simulink model "BasicAudio_TranslationEngine64"  (R2022b)
settings: Solver=FixedStepDiscrete  StartTime=0.0  StopTime=5  RelTol=1e-3  EnableMultiTasking=on
InitFcn:
  | % Initialize model
  | run([ ModelRootName() 'Init.m' ]);
  | 
  | % load library data
  | GainLibrary_data;
  | % Load saved values from partition process
  | CapturedConstMask.LoadMapFromFile(bdroot)
model workspace (MAT data in the model file):
  PreampVolumeTable_Idx : Simulink.Signal (value not decoded)
  Range : Simulink.Signal (value not decoded)
  Table_Idx : Simulink.Signal (value not decoded)
undefined symbols (not defined in the file or in its folder): Row
libraries: TuneVar x50, TOP x27, FeaturePath x7, CapturedConstLib x3
(part 2 of 4)

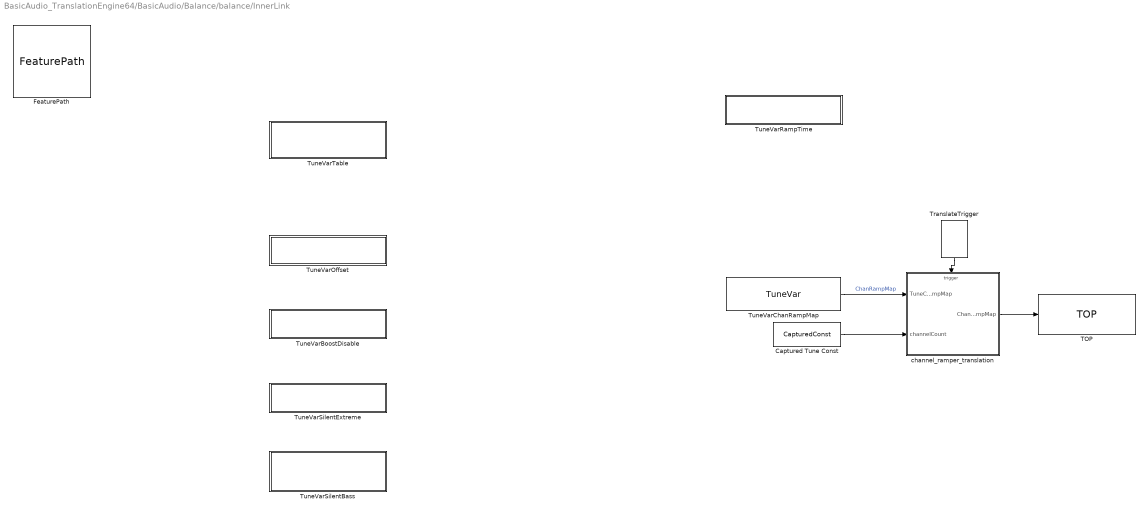
== system BasicAudio_TranslationEngine64/BasicAudio/Balance/balance/InnerLink ==
  Captured Tune Const : CapturedConstLib/CapturedConst  TriggerInit=[700 257 800 293]  Role=Automatic
      settings: SourceProductName=Bose Talaria
  FeaturePath : FeaturePath/FeaturePath  FeatureName=Balance  IsGroup=off  GroupNumber=-1  IsModule=off  TriggerInit=[-435 -186 -320 -79]
      settings: SourceProductName=Bose Talaria
  TOP : TOP/TOP  TriggerInit=[1095 215 1240 275]  TopName=ChanRampMap  DataTypeOut=single  BankNumber=0  PreOverlay=false  PostOverlay=false  CompatibilityString=[]  Role=Automatic
      settings: SourceProductName=Bose Talaria
  TranslateTrigger : TuneVar/TranslateTrigger  TriggerInit=[951 105 989 160]
      settings: SourceProductName=Bose Talaria
  TuneVarBoostDisable : Subsystem  Description=Specifies the 'boost' value to be applied to the channels towards which the balance is moved. A value of '1' indicates no 'boost' (0 dB) ,whereas '0' indicates that the 'boost' must be computed from the 'cut' value (which gets computed from the Balance table). In order to preserve the overall energy, the following formula is used: Boost^2 + Cut^2 = 2.  mask(Talaria Trivial Tune TOP){TriggerInit=[-50 240 120 280], TopName=BoostDisable, TuneName=BoostDisable, DataTypeOut=single, MaskValue=Config.DefaultMaskBoostDisable, TunabilityNumber=2, MinValue=[], MaxValue=[], BankNumber=Config.BankNumber, PreOverlay=false, PostOverlay=false, UseSameName=on}
      mask prompts: TriggerInit "Hidden: MoveFcn redraw"; TopName "Name:"; TuneName "Name of TuneVar:"; DataTypeOut "Data type:"; MaskValue "Default Value:"; TunabilityNumber "Tunability:"; MinValue "Min Value:"; MaxValue "Max Value:"; BankNumber "Target memory bank number:"; PreOverlay "Requires pre-overlay action:"; PostOverlay "Requires post-overlay action:"; UseSameName "Use same name for tune variable and TOP"
      mask help: The TuneTOP block encapsultes a Target Overlay Parameter, a Tune Variable, and a Trivial Translation between them.
      mask init:
      | [ok,activeTopPath,activeTunePath] = TuneTOP_Mask.Init(gcbh);
      settings: MoveFcn=TuneTOP_Mask.CB_TriggerInit(gcbh);
      mask Callback TriggerInit: TuneTOP_Mask.CB_TriggerInit(gcbh);
      mask TypeOptions TopName: TOP/TopName
      mask TypeOptions TuneName: Tune Variable/TuneName
      mask TypeOptions DataTypeOut: TOP/DataTypeOut
      mask TypeOptions MaskValue: Tune Variable/MaskValue
      mask TypeOptions TunabilityNumber: Tune Variable/TunabilityNumber
      mask Callback TunabilityNumber: TuneVarMask.CB_TunabilityNumber(gcbh);
      mask TypeOptions MinValue: Tune Variable/MinValue
      mask TypeOptions MaxValue: Tune Variable/MaxValue
      mask TypeOptions BankNumber: TOP/BankNumber
      mask TypeOptions PreOverlay: TOP/PreOverlay
      mask TypeOptions PostOverlay: TOP/PostOverlay
      mask Callback UseSameName: TuneTOP_Mask.CB_UseSameName(gcbh);
      mask DialogControl toolPanel Prompt: Tuning Tool Hints
      mask DialogControl DescriptionGroup Prompt: Description
      mask DialogControl EditDescription Prompt: Edit Description
      mask DialogControl EditDescription Callback: TuneTOP_Mask.CB_EditDescription(gcbh);
      mask DialogControl TunabilityText Prompt: Easy: Changes nearly every tuning.
      mask DialogControl AdvancedPanel Prompt: Advanced
      mask DialogControl ConvertToFullTranslation Prompt: Irreversible conversion to full translation
      mask DialogControl ConvertToFullTranslation Callback: TuneTOP_Mask.CB_ConvertToFullTranslation(gcbh);
      mask DialogControl ErrorContainer Prompt: Error Messages
      mask Display:
      | % retrieve icon definition
      | [path,w,h] = TuneTOP_Mask.Icon();
      | 
      | % retrieve the block's pixel size
      | pos = get(gcbh,'position');
      | bw = pos(3) - pos(1);
      | bh = pos(4) - pos(2);
      | 
      | % draw centered icon
      | xAdj = bw/2 - w/2 + 5;
      | yAdj = bh/2 - h/2 + 4;
      | for i=1:length(path)
      | 	patch(path(i).x+xAdj, path(i).y+yAdj, path(i).rgb);
      | end
      | 
      | % show the top name or an X
      | if (exist('ok','var') && ok)
      | 	text(bw*0.5, bh*0.2, activeTopPath, 'horizontalAlignment', 'center');
      | 	patch(0,0,[1 1 1]);
      | 	patch(bw,bh,[1 1 1]);
      | else
      | 	tx=bw*0.03;
      | 	ty=bh*0.03;
      | 	patch([0 tx bw bw-tx], [ty 0 bh-ty bh], [1 0 0]);
      | 	patch([0 bw-tx bw tx], [bh-ty 0 ty bh], [1 0 0]);
      | end
  TuneVarChanRampMap : TuneVar/TuneVar  Description=|  TuneName=ChanRampMap  SpecifyMaxSize=off  VariableDim=1 (Row)  MaxSize=[1 1]  TunabilityNumber=2  MinValue=[]  MaxValue=[]  TriggerInit=[630 190 800 240]  MaskValue=Config.DefaultMaskChanRampMap
      | Specifies the ramper to which each channel is mapped. Replace the channel number with:
      | '1' - 'Right'; '2' - 'Left'; '3' - 'Center'. Currently, the 'Center' group is assigned a linear gain of 1.
      settings: SourceProductName=Bose Talaria
  TuneVarOffset : Subsystem  Description=Defines the index at which the Balance is at the center i.e., neither towards the left or right sides.  mask(Talaria Trivial Tune TOP){TriggerInit=[-50 130 120 170], TopName=Offset, TuneName=Offset, DataTypeOut=single, MaskValue=Config.DefaultMaskOffset, TunabilityNumber=3, MinValue=[], MaxValue=[], BankNumber=Config.BankNumber, PreOverlay=false, PostOverlay=false, UseSameName=on}
      mask prompts: TriggerInit "Hidden: MoveFcn redraw"; TopName "Name:"; TuneName "Name of TuneVar:"; DataTypeOut "Data type:"; MaskValue "Default Value:"; TunabilityNumber "Tunability:"; MinValue "Min Value:"; MaxValue "Max Value:"; BankNumber "Target memory bank number:"; PreOverlay "Requires pre-overlay action:"; PostOverlay "Requires post-overlay action:"; UseSameName "Use same name for tune variable and TOP"
      mask help: The TuneTOP block encapsultes a Target Overlay Parameter, a Tune Variable, and a Trivial Translation between them.
      mask init:
      | [ok,activeTopPath,activeTunePath] = TuneTOP_Mask.Init(gcbh);
      settings: MoveFcn=TuneTOP_Mask.CB_TriggerInit(gcbh);
      mask Callback TriggerInit: TuneTOP_Mask.CB_TriggerInit(gcbh);
      mask TypeOptions TopName: TOP/TopName
      mask TypeOptions TuneName: Tune Variable/TuneName
      mask TypeOptions DataTypeOut: TOP/DataTypeOut
      mask TypeOptions MaskValue: Tune Variable/MaskValue
      mask TypeOptions TunabilityNumber: Tune Variable/TunabilityNumber
      mask Callback TunabilityNumber: TuneVarMask.CB_TunabilityNumber(gcbh);
      mask TypeOptions MinValue: Tune Variable/MinValue
      mask TypeOptions MaxValue: Tune Variable/MaxValue
      mask TypeOptions BankNumber: TOP/BankNumber
      mask TypeOptions PreOverlay: TOP/PreOverlay
      mask TypeOptions PostOverlay: TOP/PostOverlay
      mask Callback UseSameName: TuneTOP_Mask.CB_UseSameName(gcbh);
      mask DialogControl toolPanel Prompt: Tuning Tool Hints
      mask DialogControl DescriptionGroup Prompt: Description
      mask DialogControl EditDescription Prompt: Edit Description
      mask DialogControl EditDescription Callback: TuneTOP_Mask.CB_EditDescription(gcbh);
      mask DialogControl TunabilityText Prompt: Easy: Changes nearly every tuning.
      mask DialogControl AdvancedPanel Prompt: Advanced
      mask DialogControl ConvertToFullTranslation Prompt: Irreversible conversion to full translation
      mask DialogControl ConvertToFullTranslation Callback: TuneTOP_Mask.CB_ConvertToFullTranslation(gcbh);
      mask DialogControl ErrorContainer Prompt: Error Messages
      mask Display:
      | % retrieve icon definition
      | [path,w,h] = TuneTOP_Mask.Icon();
      | 
      | % retrieve the block's pixel size
      | pos = get(gcbh,'position');
      | bw = pos(3) - pos(1);
      | bh = pos(4) - pos(2);
      | 
      | % draw centered icon
      | xAdj = bw/2 - w/2 + 5;
      | yAdj = bh/2 - h/2 + 4;
      | for i=1:length(path)
      | 	patch(path(i).x+xAdj, path(i).y+yAdj, path(i).rgb);
      | end
      | 
      | % show the top name or an X
      | if (exist('ok','var') && ok)
      | 	text(bw*0.5, bh*0.2, activeTopPath, 'horizontalAlignment', 'center');
      | 	patch(0,0,[1 1 1]);
      | 	patch(bw,bh,[1 1 1]);
      | else
      | 	tx=bw*0.03;
      | 	ty=bh*0.03;
      | 	patch([0 tx bw bw-tx], [ty 0 bh-ty bh], [1 0 0]);
      | 	patch([0 bw-tx bw tx], [bh-ty 0 ty bh], [1 0 0]);
      | end
  TuneVarRampTime : Subsystem  Description=Specifies the default ramp time for the rampers.  mask(Talaria Trivial Tune TOP){TriggerInit=[630 -80 800 -40], TopName=RampTime, TuneName=RampTime, DataTypeOut=single, MaskValue=30, TunabilityNumber=2, MinValue=[], MaxValue=[], BankNumber=Config.BankNumber, PreOverlay=false, PostOverlay=false, UseSameName=on}
      mask prompts: TriggerInit "Hidden: MoveFcn redraw"; TopName "Name:"; TuneName "Name of TuneVar:"; DataTypeOut "Data type:"; MaskValue "Default Value:"; TunabilityNumber "Tunability:"; MinValue "Min Value:"; MaxValue "Max Value:"; BankNumber "Target memory bank number:"; PreOverlay "Requires pre-overlay action:"; PostOverlay "Requires post-overlay action:"; UseSameName "Use same name for tune variable and TOP"
      mask help: The TuneTOP block encapsultes a Target Overlay Parameter, a Tune Variable, and a Trivial Translation between them.
      mask init:
      | [ok,activeTopPath,activeTunePath] = TuneTOP_Mask.Init(gcbh);
      settings: MoveFcn=TuneTOP_Mask.CB_TriggerInit(gcbh);
      mask Callback TriggerInit: TuneTOP_Mask.CB_TriggerInit(gcbh);
      mask TypeOptions TopName: TOP/TopName
      mask TypeOptions TuneName: Tune Variable/TuneName
      mask TypeOptions DataTypeOut: TOP/DataTypeOut
      mask TypeOptions MaskValue: Tune Variable/MaskValue
      mask TypeOptions TunabilityNumber: Tune Variable/TunabilityNumber
      mask Callback TunabilityNumber: TuneVarMask.CB_TunabilityNumber(gcbh);
      mask TypeOptions MinValue: Tune Variable/MinValue
      mask TypeOptions MaxValue: Tune Variable/MaxValue
      mask TypeOptions BankNumber: TOP/BankNumber
      mask TypeOptions PreOverlay: TOP/PreOverlay
      mask TypeOptions PostOverlay: TOP/PostOverlay
      mask Callback UseSameName: TuneTOP_Mask.CB_UseSameName(gcbh);
      mask DialogControl toolPanel Prompt: Tuning Tool Hints
      mask DialogControl DescriptionGroup Prompt: Description
      mask DialogControl EditDescription Prompt: Edit Description
      mask DialogControl EditDescription Callback: TuneTOP_Mask.CB_EditDescription(gcbh);
      mask DialogControl TunabilityText Prompt: Easy: Changes nearly every tuning.
      mask DialogControl AdvancedPanel Prompt: Advanced
      mask DialogControl ConvertToFullTranslation Prompt: Irreversible conversion to full translation
      mask DialogControl ConvertToFullTranslation Callback: TuneTOP_Mask.CB_ConvertToFullTranslation(gcbh);
      mask DialogControl ErrorContainer Prompt: Error Messages
      mask Display:
      | % retrieve icon definition
      | [path,w,h] = TuneTOP_Mask.Icon();
      | 
      | % retrieve the block's pixel size
      | pos = get(gcbh,'position');
      | bw = pos(3) - pos(1);
      | bh = pos(4) - pos(2);
      | 
      | % draw centered icon
      | xAdj = bw/2 - w/2 + 5;
      | yAdj = bh/2 - h/2 + 4;
      | for i=1:length(path)
      | 	patch(path(i).x+xAdj, path(i).y+yAdj, path(i).rgb);
      | end
      | 
      | % show the top name or an X
      | if (exist('ok','var') && ok)
      | 	text(bw*0.5, bh*0.2, activeTopPath, 'horizontalAlignment', 'center');
      | 	patch(0,0,[1 1 1]);
      | 	patch(bw,bh,[1 1 1]);
      | else
      | 	tx=bw*0.03;
      | 	ty=bh*0.03;
      | 	patch([0 tx bw bw-tx], [ty 0 bh-ty bh], [1 0 0]);
      | 	patch([0 bw-tx bw tx], [bh-ty 0 ty bh], [1 0 0]);
      | end
  TuneVarSilentBass : Subsystem  mask(Talaria Trivial Tune TOP){TriggerInit=[-50 452 120 508], TopName=SleepingBeautyMutesBass, TuneName=SleepingBeautyMutesBass, DataTypeOut=single, MaskValue=Config.DefaultMaskSilentExtremeBass, TunabilityNumber=1, MinValue=[], MaxValue=[], BankNumber=Config.BankNumber, PreOverlay=false, PostOverlay=false, UseSameName=on}
      mask prompts: TriggerInit "Hidden: MoveFcn redraw"; TopName "Name:"; TuneName "Name of TuneVar:"; DataTypeOut "Data type:"; MaskValue "Default Value:"; TunabilityNumber "Tunability:"; MinValue "Min Value:"; MaxValue "Max Value:"; BankNumber "Target memory bank number:"; PreOverlay "Requires pre-overlay action:"; PostOverlay "Requires post-overlay action:"; UseSameName "Use same name for tune variable and TOP"
      mask help: The TuneTOP block encapsultes a Target Overlay Parameter, a Tune Variable, and a Trivial Translation between them.
      mask init:
      | [ok,activeTopPath,activeTunePath] = TuneTOP_Mask.Init(gcbh);
      settings: MoveFcn=TuneTOP_Mask.CB_TriggerInit(gcbh);
      mask Callback TriggerInit: TuneTOP_Mask.CB_TriggerInit(gcbh);
      mask TypeOptions TopName: TOP/TopName
      mask TypeOptions TuneName: Tune Variable/TuneName
      mask TypeOptions DataTypeOut: TOP/DataTypeOut
      mask TypeOptions MaskValue: Tune Variable/MaskValue
      mask TypeOptions TunabilityNumber: Tune Variable/TunabilityNumber
      mask Callback TunabilityNumber: TuneVarMask.CB_TunabilityNumber(gcbh);
      mask TypeOptions MinValue: Tune Variable/MinValue
      mask TypeOptions MaxValue: Tune Variable/MaxValue
      mask TypeOptions BankNumber: TOP/BankNumber
      mask TypeOptions PreOverlay: TOP/PreOverlay
      mask TypeOptions PostOverlay: TOP/PostOverlay
      mask Callback UseSameName: TuneTOP_Mask.CB_UseSameName(gcbh);
      mask DialogControl toolPanel Prompt: Tuning Tool Hints
      mask DialogControl DescriptionGroup Prompt: Description
      mask DialogControl EditDescription Prompt: Edit Description
      mask DialogControl EditDescription Callback: TuneTOP_Mask.CB_EditDescription(gcbh);
      mask DialogControl TunabilityText Prompt: Easy: Changes nearly every tuning.
      mask DialogControl AdvancedPanel Prompt: Advanced
      mask DialogControl ConvertToFullTranslation Prompt: Irreversible conversion to full translation
      mask DialogControl ConvertToFullTranslation Callback: TuneTOP_Mask.CB_ConvertToFullTranslation(gcbh);
      mask DialogControl ErrorContainer Prompt: Error Messages
      mask Display:
      | % retrieve icon definition
      | [path,w,h] = TuneTOP_Mask.Icon();
      | 
      | % retrieve the block's pixel size
      | pos = get(gcbh,'position');
      | bw = pos(3) - pos(1);
      | bh = pos(4) - pos(2);
      | 
      | % draw centered icon
      | xAdj = bw/2 - w/2 + 5;
      | yAdj = bh/2 - h/2 + 4;
      | for i=1:length(path)
      | 	patch(path(i).x+xAdj, path(i).y+yAdj, path(i).rgb);
      | end
      | 
      | % show the top name or an X
      | if (exist('ok','var') && ok)
      | 	text(bw*0.5, bh*0.2, activeTopPath, 'horizontalAlignment', 'center');
      | 	patch(0,0,[1 1 1]);
      | 	patch(bw,bh,[1 1 1]);
      | else
      | 	tx=bw*0.03;
      | 	ty=bh*0.03;
      | 	patch([0 tx bw bw-tx], [ty 0 bh-ty bh], [1 0 0]);
      | 	patch([0 bw-tx bw tx], [bh-ty 0 ty bh], [1 0 0]);
      | end
  TuneVarSilentExtreme : Subsystem  Description=|  mask(Talaria Trivial Tune TOP){TriggerInit=[-50 350 120 390], TopName=EnableSilentExtreme, TuneName=EnableSilentExtreme, DataTypeOut=single, MaskValue=Config.DefaultMaskSilentExtreme, TunabilityNumber=2, MinValue=[], MaxValue=[], BankNumber=Config.BankNumber, PreOverlay=false, PostOverlay=false, UseSameName=on}
      | 0 implies no special handling
      | 1 implies special muting of the "cut" channel, in addition to the center channels) when the input control is at its extremes (lowest or highest index is provided)
      mask prompts: TriggerInit "Hidden: MoveFcn redraw"; TopName "Name:"; TuneName "Name of TuneVar:"; DataTypeOut "Data type:"; MaskValue "Default Value:"; TunabilityNumber "Tunability:"; MinValue "Min Value:"; MaxValue "Max Value:"; BankNumber "Target memory bank number:"; PreOverlay "Requires pre-overlay action:"; PostOverlay "Requires post-overlay action:"; UseSameName "Use same name for tune variable and TOP"
      mask help: The TuneTOP block encapsultes a Target Overlay Parameter, a Tune Variable, and a Trivial Translation between them.
      mask init:
      | [ok,activeTopPath,activeTunePath] = TuneTOP_Mask.Init(gcbh);
      settings: MoveFcn=TuneTOP_Mask.CB_TriggerInit(gcbh);
      mask Callback TriggerInit: TuneTOP_Mask.CB_TriggerInit(gcbh);
      mask TypeOptions TopName: TOP/TopName
      mask TypeOptions TuneName: Tune Variable/TuneName
      mask TypeOptions DataTypeOut: TOP/DataTypeOut
      mask TypeOptions MaskValue: Tune Variable/MaskValue
      mask TypeOptions TunabilityNumber: Tune Variable/TunabilityNumber
      mask Callback TunabilityNumber: TuneVarMask.CB_TunabilityNumber(gcbh);
      mask TypeOptions MinValue: Tune Variable/MinValue
      mask TypeOptions MaxValue: Tune Variable/MaxValue
      mask TypeOptions BankNumber: TOP/BankNumber
      mask TypeOptions PreOverlay: TOP/PreOverlay
      mask TypeOptions PostOverlay: TOP/PostOverlay
      mask Callback UseSameName: TuneTOP_Mask.CB_UseSameName(gcbh);
      mask DialogControl toolPanel Prompt: Tuning Tool Hints
      mask DialogControl DescriptionGroup Prompt: Description
      mask DialogControl EditDescription Prompt: Edit Description
      mask DialogControl EditDescription Callback: TuneTOP_Mask.CB_EditDescription(gcbh);
      mask DialogControl TunabilityText Prompt: Easy: Changes nearly every tuning.
      mask DialogControl AdvancedPanel Prompt: Advanced
      mask DialogControl ConvertToFullTranslation Prompt: Irreversible conversion to full translation
      mask DialogControl ConvertToFullTranslation Callback: TuneTOP_Mask.CB_ConvertToFullTranslation(gcbh);
      mask DialogControl ErrorContainer Prompt: Error Messages
      mask Display:
      | % retrieve icon definition
      | [path,w,h] = TuneTOP_Mask.Icon();
      | 
      | % retrieve the block's pixel size
      | pos = get(gcbh,'position');
      | bw = pos(3) - pos(1);
      | bh = pos(4) - pos(2);
      | 
      | % draw centered icon
      | xAdj = bw/2 - w/2 + 5;
      | yAdj = bh/2 - h/2 + 4;
      | for i=1:length(path)
      | 	patch(path(i).x+xAdj, path(i).y+yAdj, path(i).rgb);
      | end
      | 
      | % show the top name or an X
      | if (exist('ok','var') && ok)
      | 	text(bw*0.5, bh*0.2, activeTopPath, 'horizontalAlignment', 'center');
      | 	patch(0,0,[1 1 1]);
      | 	patch(bw,bh,[1 1 1]);
      | else
      | 	tx=bw*0.03;
      | 	ty=bh*0.03;
      | 	patch([0 tx bw bw-tx], [ty 0 bh-ty bh], [1 0 0]);
      | 	patch([0 bw-tx bw tx], [bh-ty 0 ty bh], [1 0 0]);
      | end
  TuneVarTable : Subsystem  Description=Given in dB, sets the maximum impact of balance processing among channels.
  channel_ramper_translation : MATLAB Function  TreatAsAtomicUnit=on
  wires:
  Captured Tune Const/1 -> channel_ramper_translation/2(channelCount)
  TuneVarChanRampMap/1 -> channel_ramper_translation/1(TuneChanRampMap)  "ChanRampMap"
  channel_ramper_translation/1(ChanRampMap) -> TOP/1
  TranslateTrigger/1 -> channel_ramper_translation/Trigger

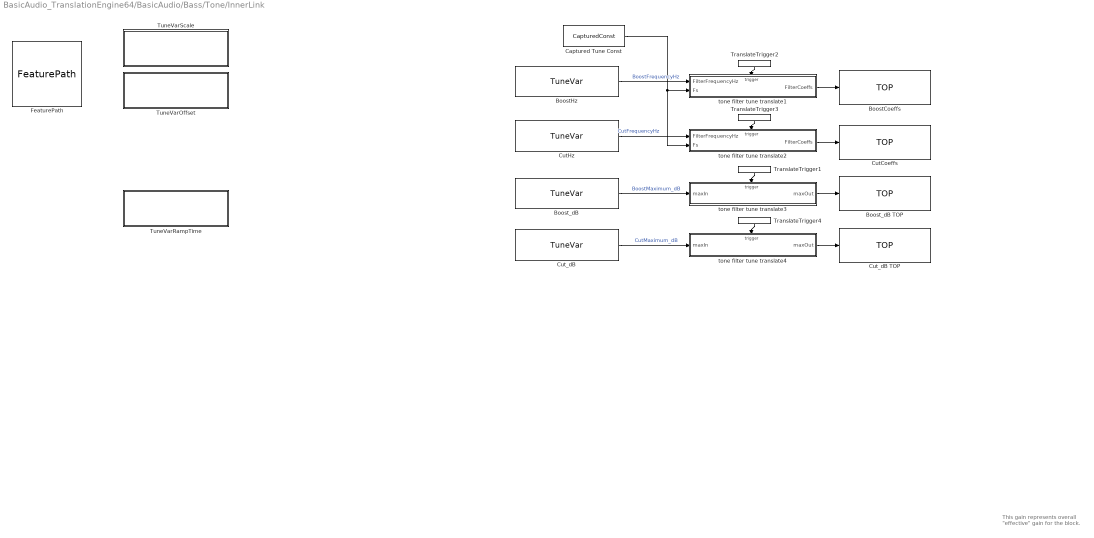
== system BasicAudio_TranslationEngine64/BasicAudio/Bass/Tone/InnerLink ==
  note: This gain represents overall
      | "effective" gain for the block.
  BoostCoeffs : TOP/TOP  TriggerInit=[-490 -218 -340 -162]  TopName=BoostCoeffs  DataTypeOut=single  BankNumber=Config.BankNumber  PreOverlay=false  PostOverlay=false  CompatibilityString=[]  Role=Automatic
      settings: SourceProductName=Bose Talaria
  BoostHz : TuneVar/TuneVar  Description=Indicates the 'corner frequency' of the target frequency band for the 'Boost' filter.  TuneName=BoostFrequencyHz  SpecifyMaxSize=off  VariableDim=1 (Row)  MaxSize=[1 1]  TunabilityNumber=1  MinValue=[]  MaxValue=[]  TriggerInit=[-1025 -225 -855 -175]  MaskValue=Config.DefaultBoostHz
      settings: SourceProductName=Bose Talaria
  Boost_dB : TuneVar/TuneVar  Description=Indicates the maximum impact in dB for the tone boost. This value must be positive. A negative boost impact would imply a gain cut instead!  TuneName=BoostMaximum_dB  SpecifyMaxSize=off  VariableDim=1 (Row)  MaxSize=[1 1]  TunabilityNumber=1  MinValue=[0]  MaxValue=[]  TriggerInit=[-1025 -40 -855 10]  MaskValue=Config.DefaultBoostDb
      settings: SourceProductName=Bose Talaria
  Boost_dB TOP : TOP/TOP  TriggerInit=[-490 -43 -340 13]  TopName=BoostMaximum_dB  DataTypeOut=single  BankNumber=Config.BankNumber  PreOverlay=false  PostOverlay=false  CompatibilityString=[]  Role=Automatic
      settings: SourceProductName=Bose Talaria
  Captured Tune Const : CapturedConstLib/CapturedConst  TriggerInit=[-945 -293 -845 -257]  Role=Automatic
      settings: SourceProductName=Bose Talaria
  CutCoeffs : TOP/TOP  TriggerInit=[-490 -128 -340 -72]  TopName=CutCoeffs  DataTypeOut=single  BankNumber=Config.BankNumber  PreOverlay=false  PostOverlay=false  CompatibilityString=[]  Role=Automatic
      settings: SourceProductName=Bose Talaria
  CutHz : TuneVar/TuneVar  Description=Indicates the 'corner frequency' of the target frequency band for the 'Cut' filter.  TuneName=CutFrequencyHz  SpecifyMaxSize=off  VariableDim=1 (Row)  MaxSize=[1 1]  TunabilityNumber=1  MinValue=[]  MaxValue=[]  TriggerInit=[-1025 -135 -855 -85]  MaskValue=Config.DefaultCutHz
      settings: SourceProductName=Bose Talaria
  Cut_dB : TuneVar/TuneVar  Description=Indicates the maximum impact in dB for the tone cut. This value must be positive. A negative cut impact would imply a gain boost instead!  TuneName=CutMaximum_dB  SpecifyMaxSize=off  VariableDim=1 (Row)  MaxSize=[1 1]  TunabilityNumber=1  MinValue=[0]  MaxValue=[]  TriggerInit=[-1025 45 -855 95]  MaskValue=Config.DefaultCutDb
      settings: SourceProductName=Bose Talaria
  Cut_dB TOP : TOP/TOP  TriggerInit=[-490 42 -340 98]  TopName=CutMaximum_dB  DataTypeOut=single  BankNumber=Config.BankNumber  PreOverlay=false  PostOverlay=false  CompatibilityString=[]  Role=Automatic
      settings: SourceProductName=Bose Talaria
  FeaturePath : FeaturePath/FeaturePath  FeatureName=Bass  IsGroup=off  GroupNumber=-1  IsModule=off  TriggerInit=[-1855 -266 -1740 -159]
      settings: SourceProductName=Bose Talaria
  TranslateTrigger1 : TuneVar/TranslateTrigger  TriggerInit=[-657 -60 -603 -50]
      settings: SourceProductName=Bose Talaria
  TranslateTrigger2 : TuneVar/TranslateTrigger  TriggerInit=[-657 -235 -603 -225]
      settings: SourceProductName=Bose Talaria
  TranslateTrigger3 : TuneVar/TranslateTrigger  TriggerInit=[-657 -145 -603 -135]
      settings: SourceProductName=Bose Talaria
  TranslateTrigger4 : TuneVar/TranslateTrigger  TriggerInit=[-657 25 -603 35]
      settings: SourceProductName=Bose Talaria
  TuneVarOffset : Subsystem  Description=Offset represents the midpoint of the index range, which separates the 'boost' indices from the 'cut' indices.  mask(Talaria Trivial Tune TOP){TriggerInit=[-1670 -213 -1500 -157], TopName=Offset, TuneName=Offset, DataTypeOut=single, MaskValue=Config.DefaultOffset, TunabilityNumber=1, MinValue=[], MaxValue=[], BankNumber=Config.BankNumber, PreOverlay=false, PostOverlay=false, UseSameName=on}
      mask prompts: TriggerInit "Hidden: MoveFcn redraw"; TopName "Name:"; TuneName "Name of TuneVar:"; DataTypeOut "Data type:"; MaskValue "Default Value:"; TunabilityNumber "Tunability:"; MinValue "Min Value:"; MaxValue "Max Value:"; BankNumber "Target memory bank number:"; PreOverlay "Requires pre-overlay action:"; PostOverlay "Requires post-overlay action:"; UseSameName "Use same name for tune variable and TOP"
      mask help: The TuneTOP block encapsultes a Target Overlay Parameter, a Tune Variable, and a Trivial Translation between them.
      mask init:
      | [ok,activeTopPath,activeTunePath] = TuneTOP_Mask.Init(gcbh);
      settings: MoveFcn=TuneTOP_Mask.CB_TriggerInit(gcbh);
      mask Callback TriggerInit: TuneTOP_Mask.CB_TriggerInit(gcbh);
      mask TypeOptions TopName: TOP/TopName
      mask TypeOptions TuneName: Tune Variable/TuneName
      mask TypeOptions DataTypeOut: TOP/DataTypeOut
      mask TypeOptions MaskValue: Tune Variable/MaskValue
      mask TypeOptions TunabilityNumber: Tune Variable/TunabilityNumber
      mask Callback TunabilityNumber: TuneVarMask.CB_TunabilityNumber(gcbh);
      mask TypeOptions MinValue: Tune Variable/MinValue
      mask TypeOptions MaxValue: Tune Variable/MaxValue
      mask TypeOptions BankNumber: TOP/BankNumber
      mask TypeOptions PreOverlay: TOP/PreOverlay
      mask TypeOptions PostOverlay: TOP/PostOverlay
      mask Callback UseSameName: TuneTOP_Mask.CB_UseSameName(gcbh);
      mask DialogControl toolPanel Prompt: Tuning Tool Hints
      mask DialogControl DescriptionGroup Prompt: Description
      mask DialogControl EditDescription Prompt: Edit Description
      mask DialogControl EditDescription Callback: TuneTOP_Mask.CB_EditDescription(gcbh);
      mask DialogControl TunabilityText Prompt: Easy: Changes nearly every tuning.
      mask DialogControl AdvancedPanel Prompt: Advanced
      mask DialogControl ConvertToFullTranslation Prompt: Irreversible conversion to full translation
      mask DialogControl ConvertToFullTranslation Callback: TuneTOP_Mask.CB_ConvertToFullTranslation(gcbh);
      mask DialogControl ErrorContainer Prompt: Error Messages
      mask Display:
      | % retrieve icon definition
      | [path,w,h] = TuneTOP_Mask.Icon();
      | 
      | % retrieve the block's pixel size
      | pos = get(gcbh,'position');
      | bw = pos(3) - pos(1);
      | bh = pos(4) - pos(2);
      | 
      | % draw centered icon
      | xAdj = bw/2 - w/2 + 5;
      | yAdj = bh/2 - h/2 + 4;
      | for i=1:length(path)
      | 	patch(path(i).x+xAdj, path(i).y+yAdj, path(i).rgb);
      | end
      | 
      | % show the top name or an X
      | if (exist('ok','var') && ok)
      | 	text(bw*0.5, bh*0.2, activeTopPath, 'horizontalAlignment', 'center');
      | 	patch(0,0,[1 1 1]);
      | 	patch(bw,bh,[1 1 1]);
      | else
      | 	tx=bw*0.03;
      | 	ty=bh*0.03;
      | 	patch([0 tx bw bw-tx], [ty 0 bh-ty bh], [1 0 0]);
      | 	patch([0 bw-tx bw tx], [bh-ty 0 ty bh], [1 0 0]);
      | end
  TuneVarRampTime : Subsystem  Description=This is the default ramp time that will be used if the RTC message has a '0' for both ramp time and ramp rate.  mask(Talaria Trivial Tune TOP){TriggerInit=[-1670 -18 -1500 38], TopName=ramptime, TuneName=ramptime, DataTypeOut=single, MaskValue=30, TunabilityNumber=1, MinValue=1, MaxValue=100000, BankNumber=0, PreOverlay=false, PostOverlay=false, UseSameName=on}
      mask prompts: TriggerInit "Hidden: MoveFcn redraw"; TopName "Name:"; TuneName "Name of TuneVar:"; DataTypeOut "Data type:"; MaskValue "Default Value:"; TunabilityNumber "Tunability:"; MinValue "Min Value:"; MaxValue "Max Value:"; BankNumber "Target memory bank number:"; PreOverlay "Requires pre-overlay action:"; PostOverlay "Requires post-overlay action:"; UseSameName "Use same name for tune variable and TOP"
      mask help: The TuneTOP block encapsultes a Target Overlay Parameter, a Tune Variable, and a Trivial Translation between them.
      mask init:
      | [ok,activeTopPath,activeTunePath] = TuneTOP_Mask.Init(gcbh);
      settings: MoveFcn=TuneTOP_Mask.CB_TriggerInit(gcbh);
      mask Callback TriggerInit: TuneTOP_Mask.CB_TriggerInit(gcbh);
      mask TypeOptions TopName: TOP/TopName
      mask TypeOptions TuneName: Tune Variable/TuneName
      mask TypeOptions DataTypeOut: TOP/DataTypeOut
      mask TypeOptions MaskValue: Tune Variable/MaskValue
      mask TypeOptions TunabilityNumber: Tune Variable/TunabilityNumber
      mask Callback TunabilityNumber: TuneVarMask.CB_TunabilityNumber(gcbh);
      mask TypeOptions MinValue: Tune Variable/MinValue
      mask TypeOptions MaxValue: Tune Variable/MaxValue
      mask TypeOptions BankNumber: TOP/BankNumber
      mask TypeOptions PreOverlay: TOP/PreOverlay
      mask TypeOptions PostOverlay: TOP/PostOverlay
      mask Callback UseSameName: TuneTOP_Mask.CB_UseSameName(gcbh);
      mask DialogControl toolPanel Prompt: Tuning Tool Hints
      mask DialogControl DescriptionGroup Prompt: Description
      mask DialogControl EditDescription Prompt: Edit Description
      mask DialogControl EditDescription Callback: TuneTOP_Mask.CB_EditDescription(gcbh);
      mask DialogControl TunabilityText Prompt: Easy: Changes nearly every tuning.
      mask DialogControl AdvancedPanel Prompt: Advanced
      mask DialogControl ConvertToFullTranslation Prompt: Irreversible conversion to full translation
      mask DialogControl ConvertToFullTranslation Callback: TuneTOP_Mask.CB_ConvertToFullTranslation(gcbh);
      mask DialogControl ErrorContainer Prompt: Error Messages
      mask Display:
      | % retrieve icon definition
      | [path,w,h] = TuneTOP_Mask.Icon();
      | 
      | % retrieve the block's pixel size
      | pos = get(gcbh,'position');
      | bw = pos(3) - pos(1);
      | bh = pos(4) - pos(2);
      | 
      | % draw centered icon
      | xAdj = bw/2 - w/2 + 5;
      | yAdj = bh/2 - h/2 + 4;
      | for i=1:length(path)
      | 	patch(path(i).x+xAdj, path(i).y+yAdj, path(i).rgb);
      | end
      | 
      | % show the top name or an X
      | if (exist('ok','var') && ok)
      | 	text(bw*0.5, bh*0.2, activeTopPath, 'horizontalAlignment', 'center');
      | 	patch(0,0,[1 1 1]);
      | 	patch(bw,bh,[1 1 1]);
      | else
      | 	tx=bw*0.03;
      | 	ty=bh*0.03;
      | 	patch([0 tx bw bw-tx], [ty 0 bh-ty bh], [1 0 0]);
      | 	patch([0 bw-tx bw tx], [bh-ty 0 ty bh], [1 0 0]);
      | end
  TuneVarScale : Subsystem  Description=Scale is used to normalize the linear gain to a value between +/- 1. The range (0,1] represents a boost while the range [-1,0) represents a cut. We use the number of available indices in each range (mapped to gain values between [-1,1]) as the denominator for normalization, i.e. as the 'Scale'.  mask(Talaria Trivial Tune TOP){TriggerInit=[-1670 -283 -1500 -227], TopName=Scale, TuneName=Scale, DataTypeOut=single, MaskValue=Config.DefaultScale, TunabilityNumber=1, MinValue=[], MaxValue=[], BankNumber=Config.BankNumber, PreOverlay=false, PostOverlay=false, UseSameName=on}
      mask prompts: TriggerInit "Hidden: MoveFcn redraw"; TopName "Name:"; TuneName "Name of TuneVar:"; DataTypeOut "Data type:"; MaskValue "Default Value:"; TunabilityNumber "Tunability:"; MinValue "Min Value:"; MaxValue "Max Value:"; BankNumber "Target memory bank number:"; PreOverlay "Requires pre-overlay action:"; PostOverlay "Requires post-overlay action:"; UseSameName "Use same name for tune variable and TOP"
      mask help: The TuneTOP block encapsultes a Target Overlay Parameter, a Tune Variable, and a Trivial Translation between them.
      mask init:
      | [ok,activeTopPath,activeTunePath] = TuneTOP_Mask.Init(gcbh);
      settings: MoveFcn=TuneTOP_Mask.CB_TriggerInit(gcbh);
      mask Callback TriggerInit: TuneTOP_Mask.CB_TriggerInit(gcbh);
      mask TypeOptions TopName: TOP/TopName
      mask TypeOptions TuneName: Tune Variable/TuneName
      mask TypeOptions DataTypeOut: TOP/DataTypeOut
      mask TypeOptions MaskValue: Tune Variable/MaskValue
      mask TypeOptions TunabilityNumber: Tune Variable/TunabilityNumber
      mask Callback TunabilityNumber: TuneVarMask.CB_TunabilityNumber(gcbh);
      mask TypeOptions MinValue: Tune Variable/MinValue
      mask TypeOptions MaxValue: Tune Variable/MaxValue
      mask TypeOptions BankNumber: TOP/BankNumber
      mask TypeOptions PreOverlay: TOP/PreOverlay
      mask TypeOptions PostOverlay: TOP/PostOverlay
      mask Callback UseSameName: TuneTOP_Mask.CB_UseSameName(gcbh);
      mask DialogControl toolPanel Prompt: Tuning Tool Hints
      mask DialogControl DescriptionGroup Prompt: Description
      mask DialogControl EditDescription Prompt: Edit Description
      mask DialogControl EditDescription Callback: TuneTOP_Mask.CB_EditDescription(gcbh);
      mask DialogControl TunabilityText Prompt: Easy: Changes nearly every tuning.
      mask DialogControl AdvancedPanel Prompt: Advanced
      mask DialogControl ConvertToFullTranslation Prompt: Irreversible conversion to full translation
      mask DialogControl ConvertToFullTranslation Callback: TuneTOP_Mask.CB_ConvertToFullTranslation(gcbh);
      mask DialogControl ErrorContainer Prompt: Error Messages
      mask Display:
      | % retrieve icon definition
      | [path,w,h] = TuneTOP_Mask.Icon();
      | 
      | % retrieve the block's pixel size
      | pos = get(gcbh,'position');
      | bw = pos(3) - pos(1);
      | bh = pos(4) - pos(2);
      | 
      | % draw centered icon
      | xAdj = bw/2 - w/2 + 5;
      | yAdj = bh/2 - h/2 + 4;
      | for i=1:length(path)
      | 	patch(path(i).x+xAdj, path(i).y+yAdj, path(i).rgb);
      | end
      | 
      | % show the top name or an X
      | if (exist('ok','var') && ok)
      | 	text(bw*0.5, bh*0.2, activeTopPath, 'horizontalAlignment', 'center');
      | 	patch(0,0,[1 1 1]);
      | 	patch(bw,bh,[1 1 1]);
      | else
      | 	tx=bw*0.03;
      | 	ty=bh*0.03;
      | 	patch([0 tx bw bw-tx], [ty 0 bh-ty bh], [1 0 0]);
      | 	patch([0 bw-tx bw tx], [bh-ty 0 ty bh], [1 0 0]);
      | end
  tone filter tune translate1 : MATLAB Function  TreatAsAtomicUnit=on  mask{MaskFilterType=Config.FilterType}
      mask prompts: MaskFilterType "Filter type"
  tone filter tune translate2 : MATLAB Function  TreatAsAtomicUnit=on  mask{MaskFilterType=Config.FilterType}
      mask prompts: MaskFilterType "Filter type"
  tone filter tune translate3 : MATLAB Function  TreatAsAtomicUnit=on
  tone filter tune translate4 : MATLAB Function  TreatAsAtomicUnit=on
  wires:
  TranslateTrigger2/1 -> tone filter tune translate1/Trigger
  BoostHz/1 -> tone filter tune translate1/1(FilterFrequencyHz)  "BoostFrequencyHz"
  TranslateTrigger3/1 -> tone filter tune translate2/Trigger
  CutHz/1 -> tone filter tune translate2/1(FilterFrequencyHz)  "CutFrequencyHz"
  tone filter tune translate1/1(FilterCoeffs) -> BoostCoeffs/1
  tone filter tune translate2/1(FilterCoeffs) -> CutCoeffs/1
  Boost_dB/1 -> tone filter tune translate3/1(maxIn)  "BoostMaximum_dB"
  tone filter tune translate3/1(maxOut) -> Boost_dB TOP/1
  Cut_dB/1 -> tone filter tune translate4/1(maxIn)  "CutMaximum_dB"
  tone filter tune translate4/1(maxOut) -> Cut_dB TOP/1
  Captured Tune Const/1 -> tone filter tune translate2/2(Fs), tone filter tune translate1/2(Fs)
  TranslateTrigger1/1 -> tone filter tune translate3/Trigger
  TranslateTrigger4/1 -> tone filter tune translate4/Trigger

== system BasicAudio_TranslationEngine64/BasicAudio/Mute/mute/InnerLink ==
  MuteControl : Subsystem  mask(Blocklib MuteControl){Config=Config, FeatureName=Mute}
      mask prompts: Config "MuteControlConfig"; FeatureName "Mask feature name:"
      mask help: This component is to be used in conjunction with 1 or more instances of the MuteRamper block. There is no mask for this component. It provides the control layer for Mute processing via an RTC and tune variable, muteControlRampTime.
      mask init:
      | blkh=gcbh;
      | Config=BTConfig.Assert(blkh,Config);
      | BTConfig.InitSetFeatureIfPresent(blkh,'FeatureName');
      | Config.Validate();
      | 
      | % Set boundary conditions
      | rampRateBounds = [5,50000];
      | rampTimeBounds = [1,3000];
      mask Help: If this control block is being used in a "multi-instance" manner, i.e. it is contorlling two or more MuteRamper blocks, there is an additional step that must be done. The developer must add a function-triggered subsytem containing an AND logic gate, which will combine the notification completion signals of the multiple ramper instances. The output of this subsytem must then feed the NTF_done input of the MuteControl block.
      mask Callback Config: BTConfig.CallbackHideIfPresent(gcbh,{'FeatureName'});
      mask TypeOptions FeatureName: FeaturePath/FeatureName
